simulink model "myNewMoto_steering"  (R2021a)
settings: Solver=FixedStepAuto  StartTime=0.0  StopTime=inf  FixedStep=0.05  RelTol=1e-3  EnableMultiTasking=on
PreLoadFcn:
  | Ts = 0.01;
  | Ts_wifi = 0.1;
libraries: arduinomotorcarrierlib x5, simulink x4, arduinosensorlib x2
settings Model: SimulationMode=external  ExtModeTrigDuration=2  Creator=bnewman  LastModifiedBy=danie
settings SolverCC: AlgebraicLoopSolver=TrustRegion
settings DataIOCC: ReturnWorkspaceOutputs=off
settings OptimizationCC: PassReuseOutputArgsThreshold=0  MaxStackSize=64
settings DebuggingCC: ParameterTunabilityLossMsg=error  ArithmeticOperatorsInVariantConditions=warning
settings HardwareCC: ProdBitPerPointer=32  ProdBitPerSizeT=32  ProdBitPerPtrDiffT=32  ProdLargestAtomicInteger=Long  ProdLargestAtomicFloat=Double  ProdWordSize=32  ProdHWDeviceType=ARM Compatible->ARM Cortex  UseEmbeddedCoderFeatures=off  UseSimulinkCoderFeatures=off
settings SFSimCC: SimUseLocalCustomCode=off  MATLABDynamicMemAlloc=off  CustomCodeUndefinedFunction=UseInterfaceOnly
settings RTWCC: SystemTargetFile=ert.tlc  HardwareBoard=Arduino MKR1000  TemplateMakefile=ert_default_tmf  GenerateReport=on  RTWUseLocalCustomCode=off  Toolchain=Arduino ARM  BuildConfiguration=Faster Runs  LaunchReport=on
settings CodeAppCC: ForceParamTrailComments=on  OperatorAnnotations=on
settings ERTTargetCC: ERTCustomFileBanners=off  SupportContinuousTime=on  SupportNonInlinedSFcns=on  RemoveResetFunc=off  SupportVariableSizeSignals=on  ModelStepFunctionPrototypeControlCompliant=off

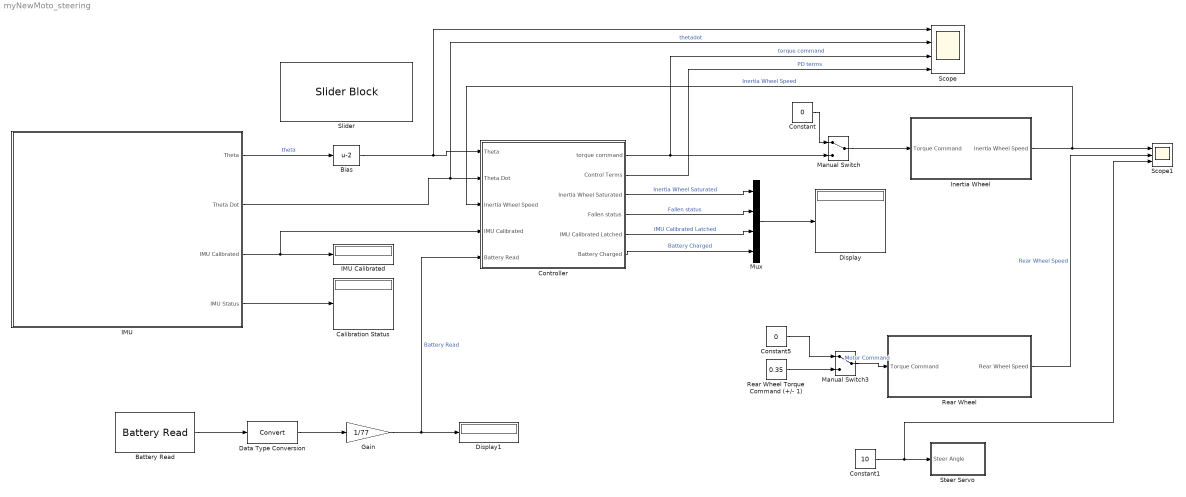
== system myNewMoto_steering ==
  Battery Read : arduinomotorcarrierlib/Battery Read  SlaveAddress=uint8( hex2dec( '66' ) )  blockPlatform=ARDUINO  SampleTime=0.05
      settings: SourceProductBaseCode=ARDUINO
  Bias : Bias  Bias=-2
  Calibration Status : Display
  Constant : Constant  Value=0
  Constant1 : Constant  Value=10
  Constant5 : Constant  Value=0
  Controller : Subsystem
  Data Type Conversion : DataTypeConversion
  Display : Display
  Display1 : Display
  Gain : Gain  Gain=1/77
  IMU : Subsystem
  IMU Calibrated : Display
  Inertia Wheel : Subsystem
  Manual Switch : ManualSwitch
  Manual Switch3 : ManualSwitch
  Mux : Mux
  Rear Wheel : Subsystem
  Rear Wheel Torque Command (+/- 1) : Constant  Value=0.35
  Scope : Scope  NumInputPorts=4
  Scope1 : Scope  NumInputPorts=3
  Slider : SliderBlock  ScaleMin=-5  ScaleMax=5
  Steer Servo : Subsystem
  wires:
  IMU/2(Theta Dot) -> Controller/2(Theta Dot), Scope/2  "thetadot"
  IMU/1(Theta) -> Bias/1  "theta"
  IMU/3(IMU Calibrated) -> Controller/4(IMU Calibrated), IMU Calibrated/1
  IMU/4(IMU Status) -> Calibration Status/1
  Controller/1(torque command) -> Scope/3, Manual Switch/2  "torque command"
  Controller/2(Control Terms) -> Scope/4  "PD terms"
  Manual Switch/1 -> Inertia Wheel/1(Torque Command)
  Constant/1 -> Manual Switch/1
  Inertia Wheel/1(Inertia Wheel Speed) -> Controller/3(Inertia Wheel Speed), Scope1/1  "Inertia Wheel Speed"
  Controller/3(Inertia Wheel Saturated) -> Mux/1  "Inertia Wheel Saturated"
  Controller/4(Fallen status) -> Mux/2  "Fallen status"
  Mux/1 -> Display/1
  Controller/5(IMU Calibrated Latched) -> Mux/3  "IMU Calibrated Latched"
  Battery Read/1 -> Data Type Conversion/1
  Data Type Conversion/1 -> Gain/1
  Gain/1 -> Controller/5(Battery Read), Display1/1  "Battery Read"
  Controller/6(Battery Charged) -> Mux/4  "Battery Charged"
  Bias/1 -> Controller/1(Theta), Scope/1
  Rear Wheel/1(Rear Wheel Speed) -> Scope1/2  "Rear Wheel Speed"
  Constant5/1 -> Manual Switch3/1
  Rear Wheel Torque Command (+/- 1)/1 -> Manual Switch3/2
  Manual Switch3/1 -> Rear Wheel/1(Torque Command)  "Motor Command"
  Constant1/1 -> Scope1/3, Steer Servo/1(Steer Angle)

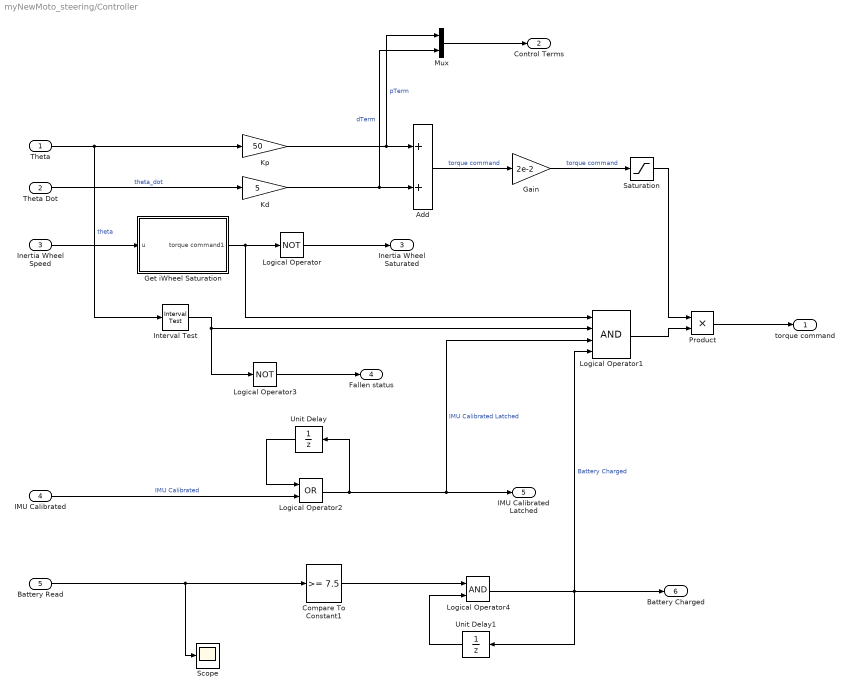
== system myNewMoto_steering/Controller ==
  Theta : Inport
  Theta Dot : Inport  Port=2
  Inertia Wheel Speed : Inport  Port=3
  IMU Calibrated : Inport  Port=4
  Battery Read : Inport  Port=5
  Add : Sum  Inputs=2
  Compare To Constant1 : simulink/Logic and Bit Operations/Compare To Constant  relop=>=  const=7.5  OutDataTypeStr=boolean
  "Gain " : Gain  Gain=2e-2
  Get iWheel Saturation : Subsystem
  Interval Test : simulink/Logic and Bit Operations/Interval Test  IntervalClosedRight=on  uplimit=6  IntervalClosedLeft=on  lowlimit=-6  OutDataTypeStr=boolean
  Kd : Gain  Gain=5
  Kp : Gain  Gain=50
  Logical Operator : Logic  Operator=NOT  AllPortsSameDT=off  OutDataTypeStr=boolean
  Logical Operator1 : Logic  Inputs=4  AllPortsSameDT=off  OutDataTypeStr=boolean
  Logical Operator2 : Logic  Operator=OR  AllPortsSameDT=off  OutDataTypeStr=boolean
  Logical Operator3 : Logic  Operator=NOT  AllPortsSameDT=off  OutDataTypeStr=boolean
  Logical Operator4 : Logic  AllPortsSameDT=off  OutDataTypeStr=boolean
  Mux : Mux  Inputs=2
  Product : Product
  Saturation : Saturate  UpperLimit=0.7  LowerLimit=-0.7
  Scope : Scope
  Unit Delay : UnitDelay  SampleTime=-1  HasFrameUpgradeWarning=on
  Unit Delay1 : UnitDelay  InitialCondition=1  SampleTime=-1  HasFrameUpgradeWarning=on
  torque command : Outport  VectorParamsAs1DForOutWhenUnconnected=off
  Control Terms : Outport  Port=2
  Inertia Wheel Saturated : Outport  Port=3  VectorParamsAs1DForOutWhenUnconnected=off
  Fallen status : Outport  Port=4  VectorParamsAs1DForOutWhenUnconnected=off
  IMU Calibrated Latched : Outport  Port=5  VectorParamsAs1DForOutWhenUnconnected=off
  Battery Charged : Outport  Port=6  VectorParamsAs1DForOutWhenUnconnected=off
  wires:
  Theta Dot/1 -> Kd/1  "theta_dot"
  Add/1 -> "Gain "/1  "torque command"
  Theta/1 -> Kp/1, Interval Test/1  "theta"
  Kd/1 -> Add/2, Mux/2  "dTerm"
  Kp/1 -> Add/1, Mux/1  "pTerm"
  "Gain "/1 -> Saturation/1  "torque command"
  Mux/1 -> Control Terms/1
  Inertia Wheel Speed/1 -> Get iWheel Saturation/1(u)
  Get iWheel Saturation/1(torque command1) -> Logical Operator1/1, Logical Operator/1
  Product/1 -> torque command/1
  Saturation/1 -> Product/1
  Logical Operator/1 -> Inertia Wheel Saturated/1
  Logical Operator1/1 -> Product/2
  Interval Test/1 -> Logical Operator1/2, Logical Operator3/1
  Logical Operator3/1 -> Fallen status/1
  Logical Operator2/1 -> IMU Calibrated Latched/1, Logical Operator1/3, Unit Delay/1  "IMU Calibrated Latched"
  Unit Delay/1 -> Logical Operator2/1
  IMU Calibrated/1 -> Logical Operator2/2  "IMU Calibrated"
  Battery Read/1 -> Scope/1, Compare To Constant1/1
  Unit Delay1/1 -> Logical Operator4/2
  Logical Operator4/1 -> Battery Charged/1, Logical Operator1/4, Unit Delay1/1  "Battery Charged"
  Compare To Constant1/1 -> Logical Operator4/1

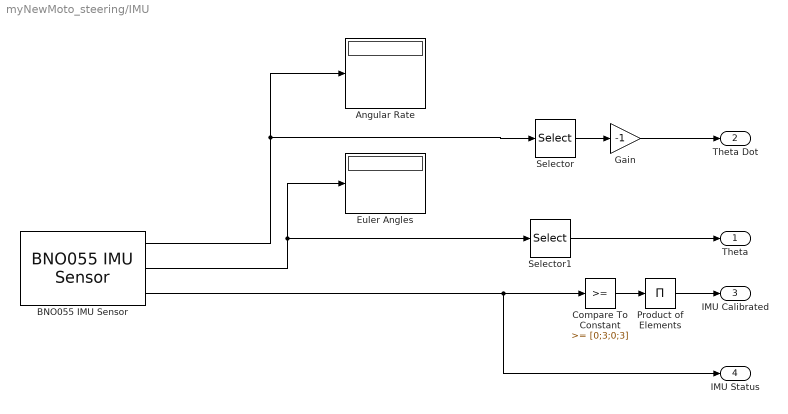
== system myNewMoto_steering/IMU ==
  Angular Rate : Display
  BNO055 IMU Sensor : arduinosensorlib/BNO055 IMU Sensor  SlaveAddress=0x28  OperationMode=Fusion  Accel=off  AngularRate=on  MagField=off  EulerAngles=on  Quat=off  LinearAccel=off  GravityVector=off  Status=on  AccelRange=4G  AccelBW=62.5 Hz  GyroRange=2000 dps  GyroBW=32 Hz  MagODR=10 Hz  SampleTime=0.05  blockPlatform=ARDUINO
      settings: SourceProductBaseCode=ARDUINO
  Compare To Constant : simulink/Logic and Bit Operations/Compare To Constant  relop=>=  const=[0;3;0;3]  OutDataTypeStr=boolean
  Euler Angles : Display
  Gain : Gain  Gain=-1
  Product of Elements : Product  Inputs=*
  Selector : Selector  InputPortWidth=3  IndexOptions=Index vector (dialog)  Indices=2  OutputSizes=1
  Selector1 : Selector  InputPortWidth=3  IndexOptions=Index vector (dialog)  Indices=2  OutputSizes=1
  Theta : Outport
  Theta Dot : Outport  Port=2
  IMU Calibrated : Outport  Port=3
  IMU Status : Outport  Port=4
  wires:
  BNO055 IMU Sensor/2 -> Euler Angles/1, Selector1/1
  BNO055 IMU Sensor/1 -> Angular Rate/1, Selector/1
  Product of Elements/1 -> IMU Calibrated/1
  BNO055 IMU Sensor/3 -> IMU Status/1, Compare To Constant/1
  Gain/1 -> Theta Dot/1
  Selector/1 -> Gain/1
  Compare To Constant/1 -> Product of Elements/1
  Selector1/1 -> Theta/1

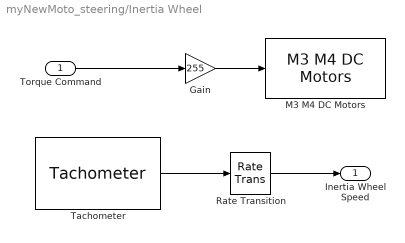
== system myNewMoto_steering/Inertia Wheel ==
  Torque Command : Inport
  Gain : Gain  Gain=255
  M3 M4 DC Motors : arduinomotorcarrierlib/M3 M4 DC Motors  MotorNumber=M3  forwardPinNumber=3  reversePinNumber=2
      settings: SourceProductBaseCode=ARDUINO
  Rate Transition : RateTransition
  Tachometer : arduinosensorlib/Tachometer  PinNumber=16  InterruptMode=RISING  PulseCountperRotation=1  SampleTime=0.1  blockPlatform=ARDUINO
      settings: SourceProductBaseCode=ARDUINO
  Inertia Wheel Speed : Outport
  wires:
  Gain/1 -> M3 M4 DC Motors/1
  Torque Command/1 -> Gain/1
  Tachometer/1 -> Rate Transition/1
  Rate Transition/1 -> Inertia Wheel Speed/1

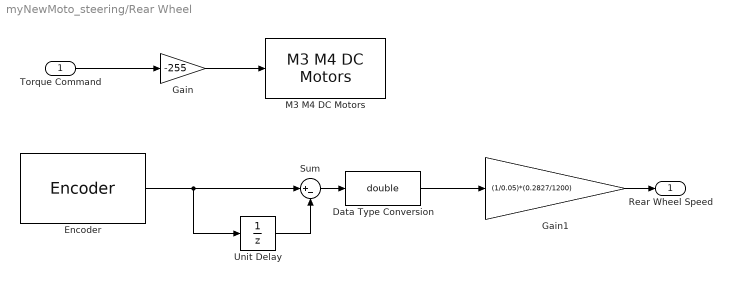
== system myNewMoto_steering/Rear Wheel ==
  Torque Command : Inport
  Data Type Conversion : DataTypeConversion  OutDataTypeStr=double
  Encoder : arduinomotorcarrierlib/Encoder  SlaveAddress=uint8( hex2dec( '66' ) )  blockPlatform=ARDUINO  Encoder=2  ShowSpeed=off  ResetOption=on  SampleTime=0.05
      settings: SourceProductBaseCode=ARDUINO
  Gain : Gain  Gain=-255
  Gain1 : Gain  Gain=(1/0.05)*(0.2827/1200)
  M3 M4 DC Motors : arduinomotorcarrierlib/M3 M4 DC Motors  MotorNumber=M4  forwardPinNumber=4  reversePinNumber=5
      settings: SourceProductBaseCode=ARDUINO
  Sum : Sum  Inputs=|+-
  Unit Delay : UnitDelay  SampleTime=-1  HasFrameUpgradeWarning=on
  Rear Wheel Speed : Outport
  wires:
  Gain/1 -> M3 M4 DC Motors/1
  Torque Command/1 -> Gain/1
  Sum/1 -> Data Type Conversion/1
  Unit Delay/1 -> Sum/2
  Data Type Conversion/1 -> Gain1/1
  Encoder/1 -> Sum/1, Unit Delay/1
  Gain1/1 -> Rear Wheel Speed/1

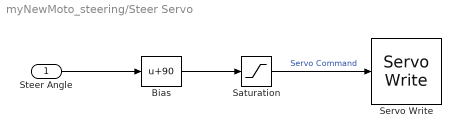
== system myNewMoto_steering/Steer Servo ==
  Steer Angle : Inport
  Bias : Bias  Bias=90
  Saturation : Saturate  UpperLimit=120  LowerLimit=60
  Servo Write : arduinomotorcarrierlib/Servo Write  SlaveAddress=uint8( hex2dec( '66' ) )  blockPlatform=ARDUINO  MotorNumber=3  MotorCarrierPWMFreq=100
      settings: SourceProductBaseCode=ARDUINO
  wires:
  Bias/1 -> Saturation/1
  Saturation/1 -> Servo Write/1  "Servo Command"
  Steer Angle/1 -> Bias/1

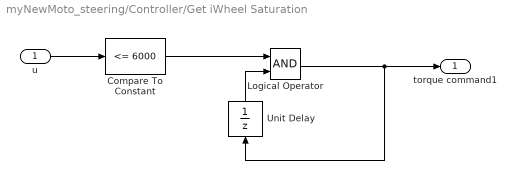
== system myNewMoto_steering/Controller/Get iWheel Saturation ==
  u : Inport
  Compare To Constant : simulink/Logic and Bit Operations/Compare To Constant  relop=<=  const=6000  OutDataTypeStr=boolean
  Logical Operator : Logic  AllPortsSameDT=off  OutDataTypeStr=boolean
  Unit Delay : UnitDelay  InitialCondition=1  SampleTime=-1  HasFrameUpgradeWarning=on
  torque command1 : Outport
  wires:
  Logical Operator/1 -> torque command1/1, Unit Delay/1
  Unit Delay/1 -> Logical Operator/2
  Compare To Constant/1 -> Logical Operator/1
  u/1 -> Compare To Constant/1
